simulink model "KF"  (R2019a)
settings: Solver=VariableStepAuto  StartTime=0.0  StopTime=10.0  RelTol=1e-3
values from neighbouring files (symbols this model uses):
  C = zeros(2,10); C(1,1) = 1; C(2,4) = 1    [parameters.m]
  GAMMA = eye(10)    [parameters.m]
  initial_P = inmat.P_ss    [parameters.m]
  initial_state = [0,0,0,0,0,0,0,0,0,0]'    [parameters.m]
  Q = XI    [augument_IP_plant.m]    (also in parameters.m = diag([XI1,XI2],0))
  R = TH    [augument_IP_plant.m]    (also in parameters.m = diag([TH1,TH2]))
undefined symbols (not defined in the file or in its folder): DELTA, PHI
settings Model: Creator=revolt  LastModifiedBy=revolt

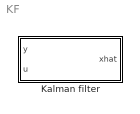
== system KF ==
  Kalman filter : Subsystem

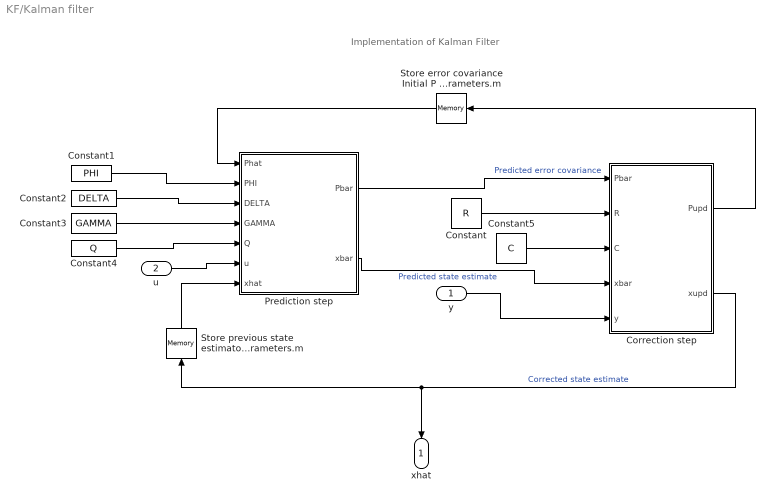
== system KF/Kalman filter ==
  note: Implementation of Kalman Filter
  y : Inport
  u : Inport  Port=2
  Constant : Constant  Value=R
  Constant1 : Constant  Value=PHI
  Constant2 : Constant  Value=DELTA
  Constant3 : Constant  Value=GAMMA
  Constant4 : Constant  Value=Q
  Constant5 : Constant  Value=C
  Correction step : MATLAB Function  TreatAsAtomicUnit=on
  Prediction step : MATLAB Function  TreatAsAtomicUnit=on
  Store error covariance Initial P set in parameters.m : Memory  InitialCondition=initial_P
  Store previous state estimaton Initial state set in parameters.m : Memory  InitialCondition=initial_state
  xhat : Outport
  wires:
  u/1 -> Prediction step/6(u)
  Store previous state estimaton Initial state set in parameters.m/1 -> Prediction step/7(xhat)
  Prediction step/2(xbar) -> Correction step/4(xbar)  "Predicted state estimate"
  Prediction step/1(Pbar) -> Correction step/1(Pbar)  "Predicted error covariance"
  Correction step/1(Pupd) -> Store error covariance Initial P set in parameters.m/1
  y/1 -> Correction step/5(y)
  Correction step/2(xupd) -> Store previous state estimaton Initial state set in parameters.m/1, xhat/1  "Corrected state estimate"
  Store error covariance Initial P set in parameters.m/1 -> Prediction step/1(Phat)
  Constant/1 -> Correction step/2(R)
  Constant1/1 -> Prediction step/2(PHI)
  Constant2/1 -> Prediction step/3(DELTA)
  Constant3/1 -> Prediction step/4(GAMMA)
  Constant4/1 -> Prediction step/5(Q)
  Constant5/1 -> Correction step/3(C)

== matlab function KF/Kalman filter/Correction step ==
  data: Pbar input; R input; C input; xbar input; Pupd output; y input; xupd output
function [Pupd, xupd] = update(Pbar,R, C,xbar,y)
% returns the mean and covariance after correcting based on the
% measurement, ref Fossen 2011 table 11.1

K = (Pbar * C')/(C * Pbar * C' + R);
xupd = xbar + K * (y - C * xbar);

I = eye(size(Pbar));
Pupd = (I - K * C) * Pbar * (I - K * C)' + K*R*K';

end

== matlab function KF/Kalman filter/Prediction step ==
  data: Pbar output; Phat input; PHI input; DELTA input; GAMMA input; Q input; u input; xhat input; xbar output
function [Pbar, xbar] = predict(Phat,PHI,DELTA,GAMMA,Q,u, xhat)
% returns the predicted mean (=state) and covariance (-covariance of 
% predicted state estimate error) for a time step Ts, ref Fossen 2011 table 11.1

% PREDICTION
xbar = PHI * xhat + DELTA * u;
Pbar = PHI * Phat * PHI' + GAMMA * Q * GAMMA';

end
